simulink model "Refined_Model_40"  (R2020b)
settings: Solver=FixedStepAuto  StartTime=0.0  StopTime=5000  FixedStep=0.1  RelTol=1e-3
values from neighbouring files (symbols this model uses):
  ALInpSpeed = AxlLoss (1,:)    [GPS_val.m]    (also in ICEBEV_Script.m; ICEBEV_Script_VECTO.m; ICE_Script.m; ICE_Script_SSVal.m)
  ALInpTor = AxlLoss(:,1)    [GPS_val.m]    (also in ICEBEV_Script.m; ICEBEV_Script_VECTO.m; ICE_Script.m; ICE_Script_SSVal.m)
  ALTableVal = AxlLoss(2:end,2:end)    [GPS_val.m]    (also in ICEBEV_Script.m; ICEBEV_Script_VECTO.m; ICE_Script.m; ICE_Script_SSVal.m)
  CovDist = RoadProfile(:,4)    [ICE_Val.m]
  Cx = VehicleDefine(7,3)    [BEV_Basictest.m]    (also in GPS_val.m; ICEBEV_Script.m; ICEBEV_Script_VECTO.m; ICE_Script.m)
  Dist = 1:length(MaxSpeedProfile)    [GPS_val.m]    (also in ICE_Script.m; ICE_Val.m = [1:CovDist(end)])
  DynRolRad = VehicleDefine(5,3)    [BEV_Basictest.m]    (also in GPS_val.m; ICEBEV_Script.m; ICEBEV_Script_VECTO.m; ICE_Script.m)
  FDR = VehicleDefine(20,3)    [BEV_Basictest.m]    (also in GPS_val.m = VehicleDefine(22,3); ICEBEV_Script.m = VehicleDefine(22,3); ICEBEV_Script_VECTO.m = VehicleDefine(22,3); ICE_Script.m = VehicleDefine(22,3))
  Fr = VehicleDefine(13,3)    [BEV_Basictest.m]    (also in GPS_val.m; ICEBEV_Script.m; ICEBEV_Script_VECTO.m; ICE_Script.m)
  g = VehicleDefine(14,3)    [BEV_Basictest.m]    (also in GPS_val.m; ICEBEV_Script.m; ICEBEV_Script_VECTO.m; ICE_Script.m)
  GNo = GBXDefine(:,1)    [GPS_val.m]    (also in ICEBEV_Script.m; ICEBEV_Script_VECTO.m; ICE_Script.m; ICE_Script_SSVal.m)
  IntpSlope = round(IntpSlope,1)    [GPS_val.m]    (also in ICE_Script.m; ICE_Val.m = A)
  Jk = VehicleDefine(15,3)    [BEV_Basictest.m]    (also in GPS_val.m; ICEBEV_Script.m; ICEBEV_Script_VECTO.m; ICE_Script.m)
  MaxAcc = 1    [BEV_Basictest.m]    (also in GPS_val.m; ICEBEV_Script.m; ICEBEV_Script_VECTO.m; ICE_Script.m)
  MaxDec = 1    [BEV_Basictest.m]    (also in GPS_val.m; ICEBEV_Script.m; ICEBEV_Script_VECTO.m; ICE_Script.m)
  MaxSpeedProfile = FMSP    [GPS_val.m]    (also in ICE_Script.m; ICE_Val.m = repelem(SegSPLatinmps,SegLeninm))
  Me = VehicleDefine(10,3)    [BEV_Basictest.m]    (also in GPS_val.m; ICEBEV_Script.m; ICEBEV_Script_VECTO.m; ICE_Script.m)
  Mt = VehicleDefine(12,3)    [BEV_Basictest.m]    (also in GPS_val.m; ICEBEV_Script.m; ICEBEV_Script_VECTO.m; ICE_Script.m)
  Mtot = Mv+Me+Mt    [BEV_Basictest.m]    (also in GPS_val.m; ICEBEV_Script.m; ICEBEV_Script_VECTO.m; ICE_Script.m)
  Mv = VehicleDefine(9,3)    [BEV_Basictest.m]    (also in GPS_val.m; ICEBEV_Script.m; ICEBEV_Script_VECTO.m; ICE_Script.m)
  NoSteps = round(Dist(end))    [GPS_val.m]    (also in ICE_Script.m; ICE_Val.m = 3002)
  NoWhlFA = VehicleDefine(2,3)    [BEV_Basictest.m]    (also in GPS_val.m; ICE_Script.m; ICE_Val.m; ICE_Val_new.m)
  NoWhlRA = VehicleDefine(4,3)    [BEV_Basictest.m]    (also in GPS_val.m; ICE_Script.m; ICE_Val.m; ICE_Val_new.m)
  rho = VehicleDefine(6,3)    [BEV_Basictest.m]    (also in GPS_val.m; ICEBEV_Script.m; ICEBEV_Script_VECTO.m; ICE_Script.m)
  s = divisors(length(MaxSpeedProfile))    [GPS_val.m]    (also in ICEBEV_Script.m = round(FLoadTor); ICEBEV_Script_VECTO.m = round(FLoadTor); ICE_Script.m = round(FLoadTor); ICE_Script_SSVal.m = round(FLoadTor))
  SegNo = RoadProfile(:,1)    [ICE_Val.m]
  SegSPLatinmps = (sqrt(aMaxLat*g*CurRadinm))    [GPS_val.m]    (also in ICE_Script.m; ICE_Val.m)
  Sx = VehicleDefine(8,3)    [BEV_Basictest.m]    (also in GPS_val.m; ICEBEV_Script.m; ICEBEV_Script_VECTO.m; ICE_Script.m)
undefined symbols (not defined in the file or in its folder): G1Inprpm, Gmot, Jgbx, Stoptimes
libraries: autolibshared x2, vehdynlibtire x2, autolibdatasheetbattery x1, autolibmappedmotor x1
(part 1 of 3)
settings Model: Creator=Kshitij  LastModifiedBy=Kshitij
settings DebuggingCC: AlgebraicLoopMsg=none

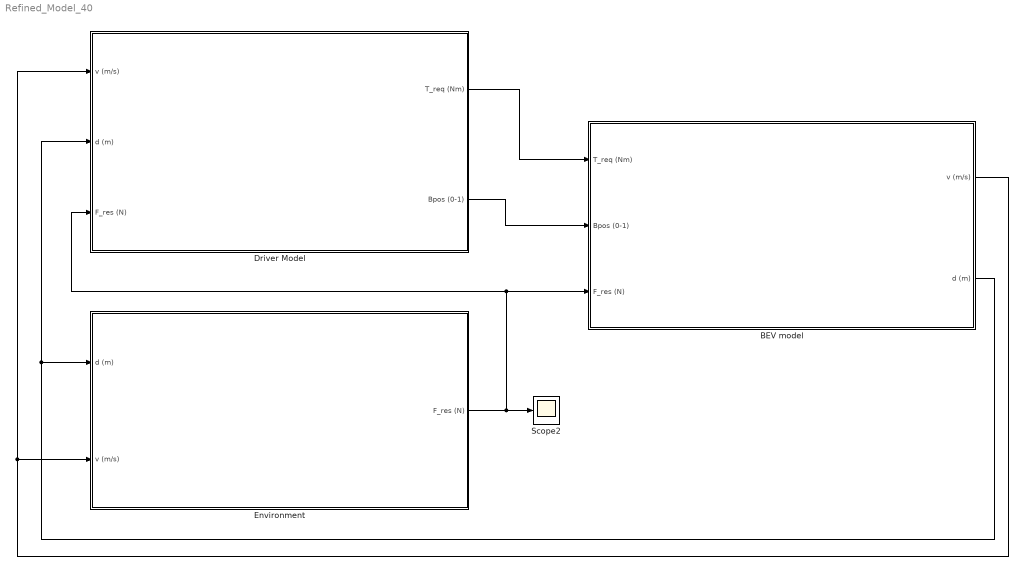
== system Refined_Model_40 ==
  BEV model : Subsystem
  Driver Model : Subsystem
  Environment : Subsystem
  Scope2 : Scope
  wires:
  Environment/1(F_res (N)) -> Driver Model/3(F_res (N)), BEV model/3(F_res (N)), Scope2/1
  Driver Model/2(Bpos (0-1)) -> BEV model/2(Bpos (0-1))
  BEV model/1(v (m/s)) -> Driver Model/1(v (m/s)), Environment/2(v (m/s))
  BEV model/2(d (m)) -> Driver Model/2(d (m)), Environment/1(d (m))
  Driver Model/1(T_req (Nm)) -> BEV model/1(T_req (Nm))

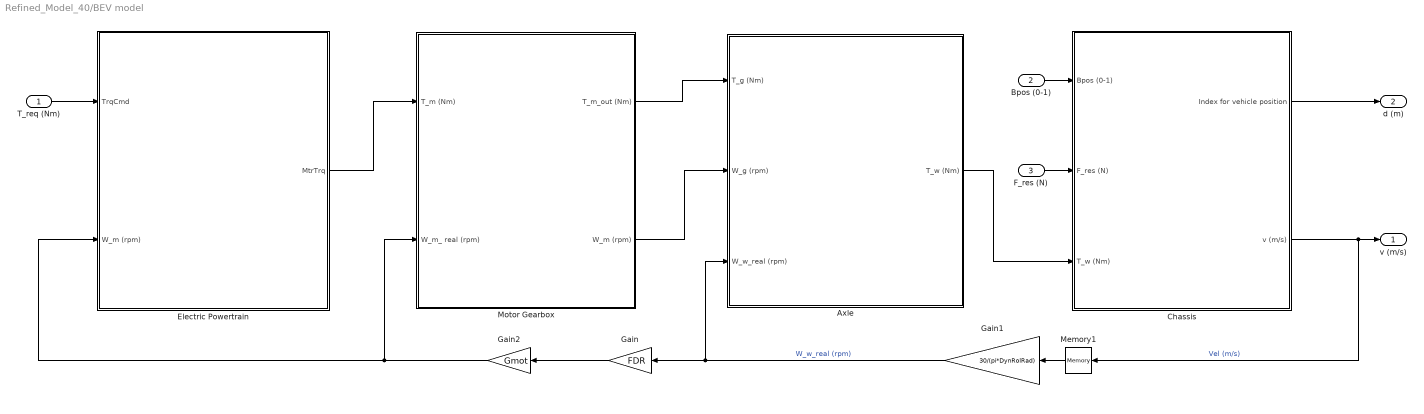
== system Refined_Model_40/BEV model ==
  T_req (Nm) : Inport
  Bpos (0-1) : Inport  Port=2
  F_res (N) : Inport  Port=3
  Axle : Subsystem
  Chassis : Subsystem
  Electric Powertrain : Subsystem
  Gain : Gain  Gain=FDR
  Gain1 : Gain  Gain=30/(pi*DynRolRad)
  Gain2 : Gain  Gain=Gmot
  Memory1 : Memory
  Motor Gearbox : Subsystem
  v (m/s) : Outport
  d (m) : Outport  Port=2
  wires:
  Motor Gearbox/2(W_m (rpm)) -> Axle/2(W_g (rpm))
  Motor Gearbox/1(T_m_out (Nm)) -> Axle/1(T_g (Nm))
  Gain1/1 -> Gain/1, Axle/3(W_w_real (rpm))  "W_w_real (rpm)"
  Chassis/2(v (m/s)) -> v (m/s)/1, Memory1/1  "Vel (m/s)"
  Axle/1(T_w (Nm)) -> Chassis/3(T_w (Nm))
  Electric Powertrain/1(MtrTrq) -> Motor Gearbox/1(T_m (Nm))
  Gain/1 -> Gain2/1
  Memory1/1 -> Gain1/1
  Bpos (0-1)/1 -> Chassis/1(Bpos (0-1))
  T_req (Nm)/1 -> Electric Powertrain/1(TrqCmd)
  F_res (N)/1 -> Chassis/2(F_res (N))
  Chassis/1(Index for vehicle position) -> d (m)/1
  Gain2/1 -> Motor Gearbox/2(W_m_ real (rpm)), Electric Powertrain/2(W_m (rpm))

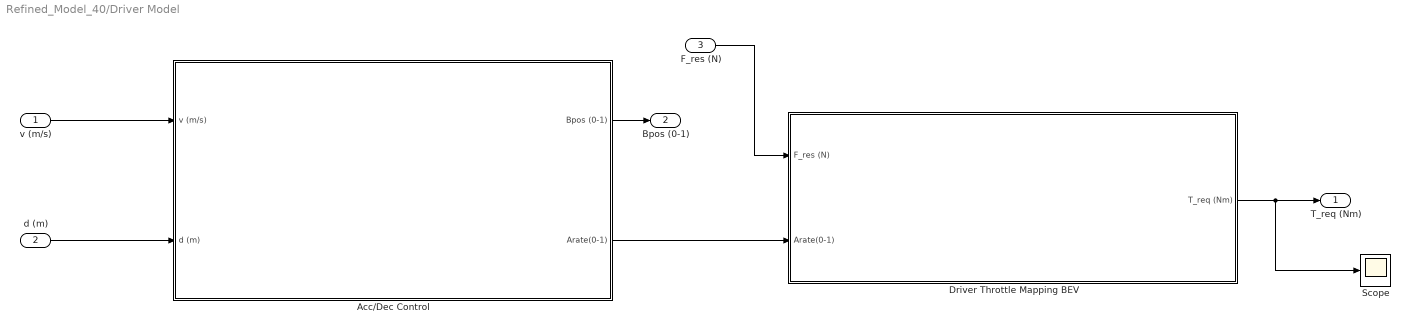
== system Refined_Model_40/Driver Model ==
  v (m/s) : Inport
  d (m) : Inport  Port=2
  F_res (N) : Inport  Port=3
  Acc/Dec Control : Subsystem
  Driver Throttle Mapping BEV : Subsystem
  Scope : Scope
  T_req (Nm) : Outport
  Bpos (0-1) : Outport  Port=2
  wires:
  Acc/Dec Control/1(Bpos (0-1)) -> Bpos (0-1)/1
  d (m)/1 -> Acc/Dec Control/2(d (m))
  F_res (N)/1 -> Driver Throttle Mapping BEV/1(F_res (N))
  Acc/Dec Control/2(Arate(0-1)) -> Driver Throttle Mapping BEV/2(Arate(0-1))
  v (m/s)/1 -> Acc/Dec Control/1(v (m/s))
  Driver Throttle Mapping BEV/1(T_req (Nm)) -> Scope/1, T_req (Nm)/1
